simulink model "teleoperation"  (R2021a)
settings: Solver=FixedStepAuto  StartTime=0.0  StopTime=10  FixedStep=0.001  RelTol=1e-3
values from neighbouring files (symbols this model uses):
  Be = 0    [four_channel_bilateral_teleoperation_architecture_params.m]    (also in params_teleop.m = 100)
  Bh = 70    [four_channel_bilateral_teleoperation_architecture_params.m]    (also in params_teleop.m)
  Bm = 0.8    [four_channel_bilateral_teleoperation_architecture_params.m]    (also in params_teleop.m)
  Bs = 0.8*4    (= 3.2)    [four_channel_bilateral_teleoperation_architecture_params.m]    (also in params_teleop.m)
  Dhst = 1000    [params_teleop.m]
  Dm = 0    [four_channel_bilateral_teleoperation_architecture_params.m]    (also in params_teleop.m)
  Ds = 0    [four_channel_bilateral_teleoperation_architecture_params.m]    (also in params_teleop.m)
  Je = 0    [four_channel_bilateral_teleoperation_architecture_params.m]    (also in params_teleop.m)
  Jh = 0.5    [four_channel_bilateral_teleoperation_architecture_params.m]    (also in params_teleop.m)
  Ke = 200    [four_channel_bilateral_teleoperation_architecture_params.m]    (also in params_teleop.m)
  Kh = 2000    [four_channel_bilateral_teleoperation_architecture_params.m]    (also in params_teleop.m)
  Khst = 20000    [params_teleop.m]
  Km = 1    [four_channel_bilateral_teleoperation_architecture_params.m]    (also in params_teleop.m)
  Ks = 4    [four_channel_bilateral_teleoperation_architecture_params.m]    (also in params_teleop.m)
  Mm = 0.5    [four_channel_bilateral_teleoperation_architecture_params.m]    (also in params_teleop.m)
  Ms = 2    [four_channel_bilateral_teleoperation_architecture_params.m]    (also in params_teleop.m)
  qe = 0.1    [params_teleop.m]
libraries: cstblocks x6
settings Model: Creator=antoninoparisi  LastModifiedBy=antoninoparisi

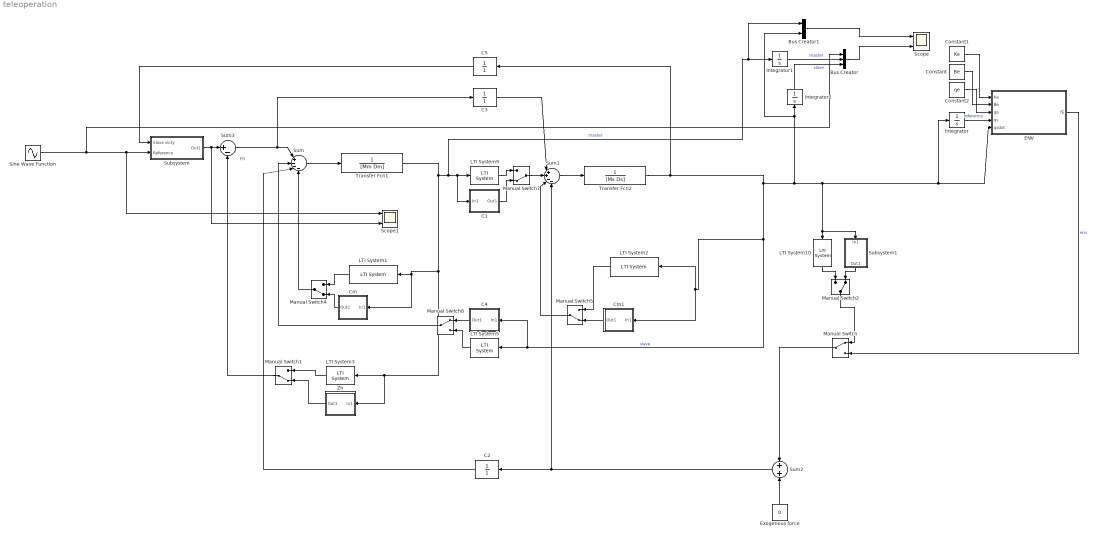
== system teleoperation ==
  note: Fh
  Bus Creator : BusCreator  Inputs=3
  Bus Creator1 : BusCreator  Inputs=2
  C1 : Subsystem
  C2 : TransferFcn  Denominator=[1]
  C3 : TransferFcn  Denominator=[1]
  C4 : Subsystem
  C5 : TransferFcn  Denominator=[1]
  Cm : Subsystem
  Cm1 : Subsystem
  Constant : Constant  Value=Be
  Constant1 : Constant  Value=Ke
  Constant2 : Constant  Value=qe
  ENV : MATLAB Function  TreatAsAtomicUnit=on
  Exogenous force : Constant  Value=0
  Integrator : Integrator
  Integrator1 : Integrator
  Integrator2 : Integrator
  LTI System1 : cstblocks/LTI System  sys=Cm  IC=[]
  LTI System10 : cstblocks/LTI System  sys=Ze  IC=[]
  LTI System2 : cstblocks/LTI System  sys=Cs  IC=[]
  LTI System3 : cstblocks/LTI System  sys=Zh  IC=[]
  LTI System5 : cstblocks/LTI System  sys=C4  IC=[]
  LTI System9 : cstblocks/LTI System  sys=C1  IC=[]
  Manual Switch : ManualSwitch
  Manual Switch{1..2,4..5,7} (5 alike) : ManualSwitch  CurrentSetting=0
  Manual Switch8 : ManualSwitch
  Scope : Scope  NumInputPorts=2
  Scope1 : Scope  NumInputPorts=3
  Sine Wave Function : Sin  Frequency=2  SampleTime=0
  Subsystem : Subsystem
  Subsystem1 : Subsystem
  Sum : Sum  Inputs=|+---
  Sum1 : Sum  Inputs=|++--
  Sum2 : Sum
  Sum3 : Sum  Inputs=|+-
  Transfer Fcn1 : TransferFcn  Denominator=[Mm Dm]
  Transfer Fcn2 : TransferFcn  Denominator=[Ms Ds]
  Zh : Subsystem
  wires:
  C2/1 -> Sum/3
  Transfer Fcn2/1 -> C5/1, Bus Creator1/2, Integrator2/1, Integrator/1, ENV/5(qsdot), Subsystem1/1(In1), LTI System10/1, C4/1(In1), LTI System5/1, LTI System2/1, Cm1/1(In1)  "slave"
  Sum1/1 -> Transfer Fcn2/1
  C3/1 -> Sum1/1
  ENV/1(fE) -> Manual Switch/2  "env"
  Constant1/1 -> ENV/1(Ke)
  Constant/1 -> ENV/2(Be)
  Constant2/1 -> ENV/3(qe)
  Sum3/1 -> C3/1, Sum/1
  Sum2/1 -> Sum1/4, C2/1
  Integrator/1 -> ENV/4(qs)  "reference"
  Manual Switch/1 -> Sum2/1
  Exogenous force/1 -> Sum2/2
  LTI System3/1 -> Manual Switch1/1
  Zh/1(Out1) -> Manual Switch1/2
  Manual Switch1/1 -> Sum3/2
  LTI System10/1 -> Manual Switch2/1
  Subsystem1/1(Out1) -> Manual Switch2/2
  Manual Switch2/1 -> Manual Switch/1
  Transfer Fcn1/1 -> LTI System1/1, Cm/1(In1), Zh/1(In1), LTI System3/1, Bus Creator1/1, Integrator1/1, C1/1(In1), LTI System9/1  "master"
  Sum/1 -> Transfer Fcn1/1
  LTI System1/1 -> Manual Switch4/1
  Cm/1(Out1) -> Manual Switch4/2
  Manual Switch4/1 -> Sum/4
  Cm1/1(Out1) -> Manual Switch5/2
  LTI System2/1 -> Manual Switch5/1
  Manual Switch5/1 -> Sum1/3
  Manual Switch7/1 -> Sum1/2
  LTI System9/1 -> Manual Switch7/1
  C1/1(Out1) -> Manual Switch7/2
  C4/1(Out1) -> Manual Switch8/1
  LTI System5/1 -> Manual Switch8/2
  Manual Switch8/1 -> Sum/2
  Bus Creator/1 -> Scope/2
  Sine Wave Function/1 -> Bus Creator/1, Scope1/1, Subsystem/2(Reference)
  Integrator2/1 -> Bus Creator/3  "slave"
  Integrator1/1 -> Bus Creator/2  "master"
  Subsystem/1(Out1) -> Sum3/1, Scope1/3
  Bus Creator1/1 -> Scope/1
  C5/1 -> Subsystem/1(Slave vlcty)

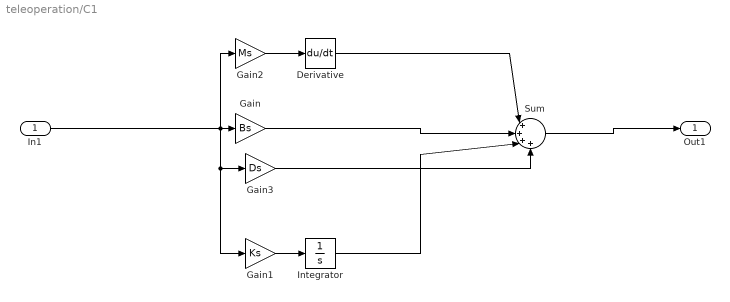
== system teleoperation/C1 ==
  In1 : Inport
  Derivative : Derivative
  Gain : Gain  Gain=Bs
  Gain1 : Gain  Gain=Ks
  Gain2 : Gain  Gain=Ms
  Gain3 : Gain  Gain=Ds
  Integrator : Integrator
  Sum : Sum  Inputs=|++++
  Out1 : Outport
  wires:
  In1/1 -> Gain3/1, Gain1/1, Gain2/1, Gain/1
  Sum/1 -> Out1/1
  Gain1/1 -> Integrator/1
  Integrator/1 -> Sum/3
  Gain/1 -> Sum/2
  Gain2/1 -> Derivative/1
  Derivative/1 -> Sum/1
  Gain3/1 -> Sum/4

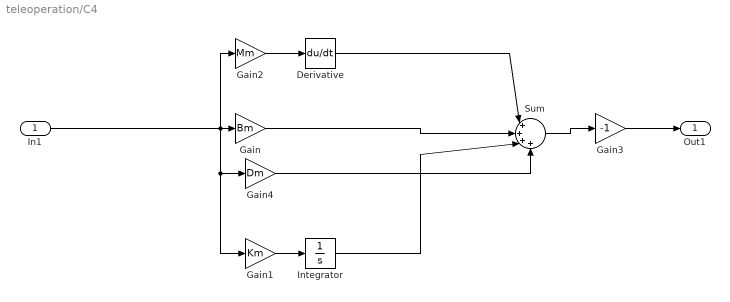
== system teleoperation/C4 ==
  In1 : Inport
  Derivative : Derivative
  Gain : Gain  Gain=Bm
  Gain1 : Gain  Gain=Km
  Gain2 : Gain  Gain=Mm
  Gain3 : Gain  Gain=-1
  Gain4 : Gain  Gain=Dm
  Integrator : Integrator
  Sum : Sum  Inputs=|++++
  Out1 : Outport
  wires:
  In1/1 -> Gain1/1, Gain4/1, Gain2/1, Gain/1
  Gain1/1 -> Integrator/1
  Integrator/1 -> Sum/3
  Gain/1 -> Sum/2
  Gain2/1 -> Derivative/1
  Derivative/1 -> Sum/1
  Gain3/1 -> Out1/1
  Sum/1 -> Gain3/1
  Gain4/1 -> Sum/4

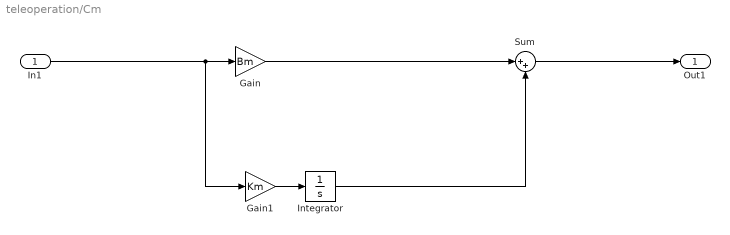
== system teleoperation/Cm ==
  In1 : Inport
  Gain : Gain  Gain=Bm
  Gain1 : Gain  Gain=Km
  Integrator : Integrator
  Sum : Sum  Inputs=|++
  Out1 : Outport
  wires:
  In1/1 -> Gain/1, Gain1/1
  Sum/1 -> Out1/1
  Gain1/1 -> Integrator/1
  Integrator/1 -> Sum/2
  Gain/1 -> Sum/1

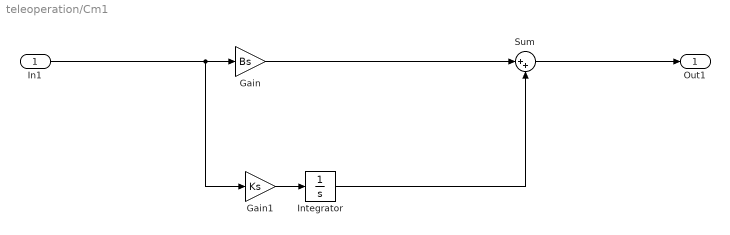
== system teleoperation/Cm1 ==
  In1 : Inport
  Gain : Gain  Gain=Bs
  Gain1 : Gain  Gain=Ks
  Integrator : Integrator
  Sum : Sum  Inputs=|++
  Out1 : Outport
  wires:
  In1/1 -> Gain/1, Gain1/1
  Sum/1 -> Out1/1
  Gain1/1 -> Integrator/1
  Integrator/1 -> Sum/2
  Gain/1 -> Sum/1

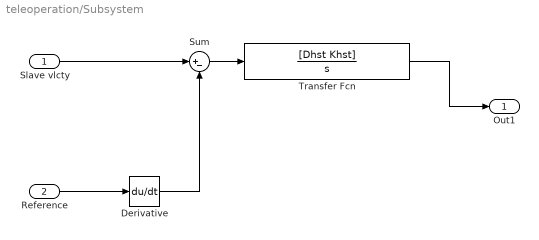
== system teleoperation/Subsystem ==
  Slave vlcty : Inport
  Reference : Inport  Port=2
  Derivative : Derivative
  Sum : Sum  Inputs=|+-
  Transfer Fcn : TransferFcn  Numerator=[Dhst Khst]  Denominator=[1 0]
  Out1 : Outport
  wires:
  Slave vlcty/1 -> Sum/1
  Sum/1 -> Transfer Fcn/1
  Transfer Fcn/1 -> Out1/1
  Reference/1 -> Derivative/1
  Derivative/1 -> Sum/2

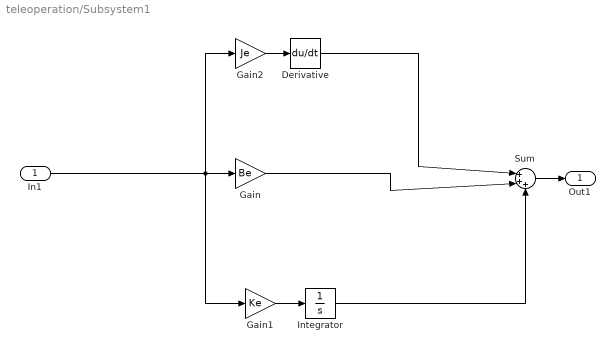
== system teleoperation/Subsystem1 ==
  In1 : Inport
  Derivative : Derivative
  Gain : Gain  Gain=Be
  Gain1 : Gain  Gain=Ke
  Gain2 : Gain  Gain=Je
  Integrator : Integrator
  Sum : Sum  Inputs=|+++
  Out1 : Outport
  wires:
  In1/1 -> Gain1/1, Gain2/1, Gain/1
  Gain2/1 -> Derivative/1
  Sum/1 -> Out1/1
  Derivative/1 -> Sum/1
  Gain/1 -> Sum/2
  Gain1/1 -> Integrator/1
  Integrator/1 -> Sum/3

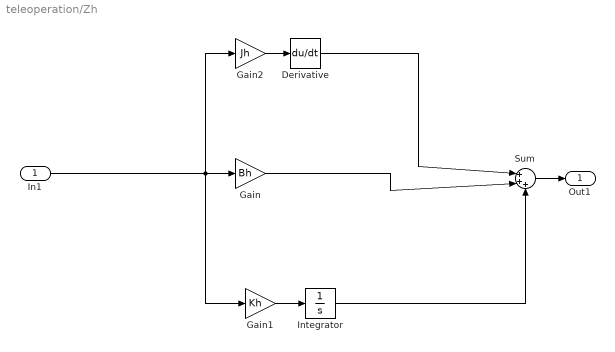
== system teleoperation/Zh ==
  In1 : Inport
  Derivative : Derivative
  Gain : Gain  Gain=Bh
  Gain1 : Gain  Gain=Kh
  Gain2 : Gain  Gain=Jh
  Integrator : Integrator
  Sum : Sum  Inputs=|+++
  Out1 : Outport
  wires:
  In1/1 -> Gain1/1, Gain2/1, Gain/1
  Gain2/1 -> Derivative/1
  Sum/1 -> Out1/1
  Derivative/1 -> Sum/1
  Gain/1 -> Sum/2
  Gain1/1 -> Integrator/1
  Integrator/1 -> Sum/3

== matlab function teleoperation/ENV ==
  data: Ke input; Be input; qe input; fE output; qs input; qsdot input
function fE = environment(Ke, Be, qe, qs, qsdot)
if(qs>qe)
fE = Ke * (qs - qe) + Be * qsdot;
else
fE = 0;
end
